simulink model "Evitar_Paredes"  (R2023b)
settings: Solver=VariableStepAuto  StartTime=0.0  StopTime=inf  RelTol=1e-3
libraries: arduinosensorlib x2
settings Model: Creator=Alberto  LastModifiedBy=Gonzalo
settings DebuggingCC: ParameterOverflowMsg=none

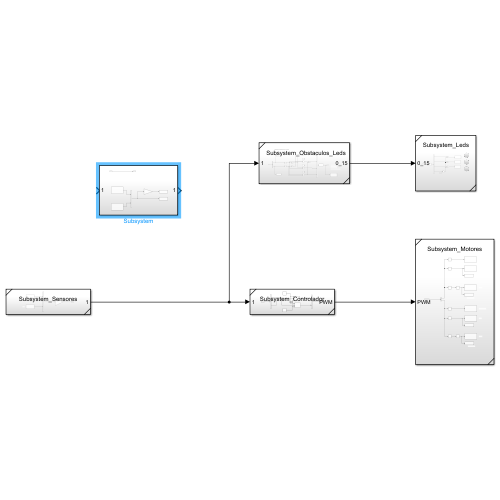
[thumbnail: Simulink's stored preview of the top-level diagram]
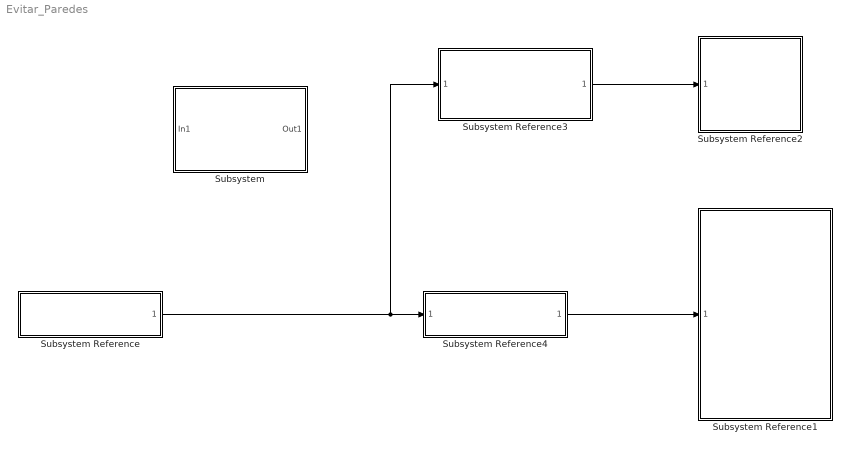
== system Evitar_Paredes ==
  Subsystem : Subsystem
  Subsystem Reference : Subsystem  ReferencedSubsystem=Subsystem_Sensores
  Subsystem Reference1 : Subsystem  ReferencedSubsystem=Subsystem_Motores
  Subsystem Reference2 : Subsystem  ReferencedSubsystem=Subsystem_Leds
  Subsystem Reference3 : Subsystem  ReferencedSubsystem=Subsystem_Obstaculos_Leds
  Subsystem Reference4 : Subsystem  ReferencedSubsystem=Subsystem_Controlador
  wires:
  Subsystem Reference/1 -> Subsystem Reference4/1, Subsystem Reference3/1
  Subsystem Reference3/1 -> Subsystem Reference2/1
  Subsystem Reference4/1 -> Subsystem Reference1/1

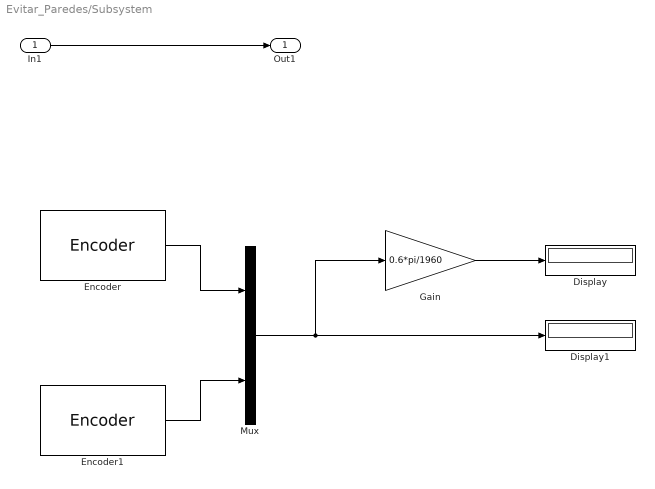
== system Evitar_Paredes/Subsystem ==
  In1 : Inport
  Display : Display
  Display1 : Display
  Encoder : arduinosensorlib/Encoder  InputA=2  InputB=3  Mode=No reset  SampleTime=-1
  Encoder1 : arduinosensorlib/Encoder  InputA=2  InputB=3  Mode=No reset  SampleTime=-1
  Gain : Gain  Gain=0.6*pi/1960
  Mux : Mux  Inputs=2
  Out1 : Outport
  wires:
  In1/1 -> Out1/1
  Encoder/1 -> Mux/1
  Encoder1/1 -> Mux/2
  Mux/1 -> Display1/1, Gain/1
  Gain/1 -> Display/1
